simulink library "BO_TYPEB_MASTER"  (Simulink 8.6)
settings: Solver=ode45  StartTime=0.0  StopTime=10.0  RelTol=1e-3
libraries: cdsEpicsBinIn x2, cdsEpicsOut x2, cdsBit2Word x2
settings Model: Creator=controls  LastModifiedBy=controls

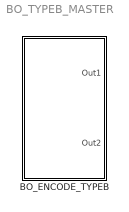
== system BO_TYPEB_MASTER ==
  BO_ENCODE_TYPEB : Subsystem

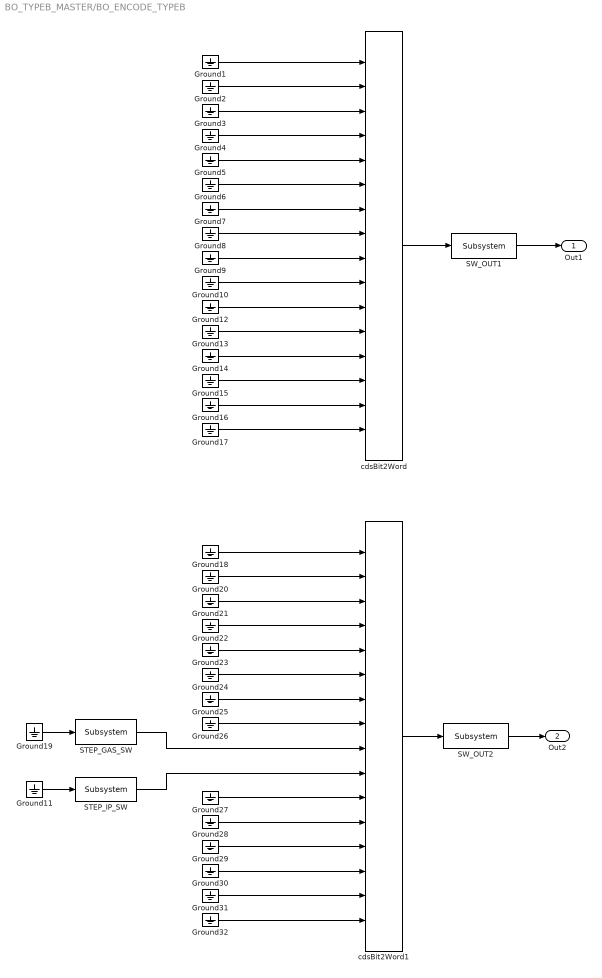
== system BO_TYPEB_MASTER/BO_ENCODE_TYPEB ==
  Ground{1..32} (32 alike) : Ground
  STEP_GAS_SW : cdsEpicsBinIn/Subsystem  Tag=cdsEpicsBinIn  Description=|
      | Purpose:                                                                            
      | Create an EPICS binary (0 or 1) input channel to the FE realtime controls.          
      |                                                                                     
      | Operation:                                                                          
      | Outputs value from an EPICS ai record. Value is binary input (bi Epics record type).
      |                                                                                     
      | Usage:                                                                              
      | Name the part with the desired EPICS channel name.
      settings: AttributesFormatString=%<Tag>
  STEP_IP_SW : cdsEpicsBinIn/Subsystem  Tag=cdsEpicsBinIn  Description=|
      | Purpose:                                                                            
      | Create an EPICS binary (0 or 1) input channel to the FE realtime controls.          
      |                                                                                     
      | Operation:                                                                          
      | Outputs value from an EPICS ai record. Value is binary input (bi Epics record type).
      |                                                                                     
      | Usage:                                                                              
      | Name the part with the desired EPICS channel name.
      settings: AttributesFormatString=%<Tag>
  SW_OUT1 : cdsEpicsOut/Subsystem  Tag=cdsEpicsOutput  Description=|
      | Purpose:                                          
      | Output a FE signal to an EPICS channel.           
      |                                                   
      | Operation:                                        
      | Takes input value and passes it to EPICS record.  
      |                                                   
      | Usage:                                            
      | Name the part with the desired EPICS rrecord name.
      settings: AttributesFormatString=%<Tag>
  SW_OUT2 : cdsEpicsOut/Subsystem  Tag=cdsEpicsOutput  Description=|
      | Purpose:                                          
      | Output a FE signal to an EPICS channel.           
      |                                                   
      | Operation:                                        
      | Takes input value and passes it to EPICS record.  
      |                                                   
      | Usage:                                            
      | Name the part with the desired EPICS rrecord name.
      settings: AttributesFormatString=%<Tag>
  cdsBit2Word : cdsBit2Word/cdsBit2Word  Tag=cdsBit2Word  Description=Forms single 16 bit integer from 16 0/1 inputs.
      settings: AttributesFormatString=%<Tag>
  cdsBit2Word1 : cdsBit2Word/cdsBit2Word  Tag=cdsBit2Word  Description=Forms single 16 bit integer from 16 0/1 inputs.
      settings: AttributesFormatString=%<Tag>
  Out1 : Outport
  Out2 : Outport  Port=2
  wires:
  STEP_GAS_SW/1 -> cdsBit2Word1/9
  STEP_IP_SW/1 -> cdsBit2Word1/10
  Ground19/1 -> STEP_GAS_SW/1
  Ground11/1 -> STEP_IP_SW/1
  cdsBit2Word1/1 -> SW_OUT2/1
  cdsBit2Word/1 -> SW_OUT1/1
  SW_OUT1/1 -> Out1/1
  SW_OUT2/1 -> Out2/1
  Ground5/1 -> cdsBit2Word/5
  Ground12/1 -> cdsBit2Word/11
  Ground14/1 -> cdsBit2Word/13
  Ground2/1 -> cdsBit2Word/2
  Ground9/1 -> cdsBit2Word/9
  Ground6/1 -> cdsBit2Word/6
  Ground1/1 -> cdsBit2Word/1
  Ground8/1 -> cdsBit2Word/8
  Ground13/1 -> cdsBit2Word/12
  Ground4/1 -> cdsBit2Word/4
  Ground7/1 -> cdsBit2Word/7
  Ground15/1 -> cdsBit2Word/14
  Ground10/1 -> cdsBit2Word/10
  Ground16/1 -> cdsBit2Word/15
  Ground17/1 -> cdsBit2Word/16
  Ground3/1 -> cdsBit2Word/3
  Ground20/1 -> cdsBit2Word1/2
  Ground22/1 -> cdsBit2Word1/4
  Ground18/1 -> cdsBit2Word1/1
  Ground21/1 -> cdsBit2Word1/3
  Ground24/1 -> cdsBit2Word1/6
  Ground26/1 -> cdsBit2Word1/8
  Ground25/1 -> cdsBit2Word1/7
  Ground23/1 -> cdsBit2Word1/5
  Ground28/1 -> cdsBit2Word1/12
  Ground31/1 -> cdsBit2Word1/15
  Ground27/1 -> cdsBit2Word1/11
  Ground32/1 -> cdsBit2Word1/16
  Ground30/1 -> cdsBit2Word1/14
  Ground29/1 -> cdsBit2Word1/13
